simulink model "vehicle_control"  (R2021b)
settings: Solver=ode1  StartTime=0.0  StopTime=Ts  FixedStep=0.01  RelTol=1e-3
values from neighbouring files (symbols this model uses):
  L = 3    [MultiAgent_initiateSAC.m]    (also in control_velocity.m; initiate.m; initiateHybrid.m; initiateSAC.m)
  ld = 5    [MultiAgent_initiateSAC.m]    (also in control_velocity.m; initiate.m = vel/2; initiateHybrid.m; initiateSAC.m)
  psi_o = 0    [MultiAgent_initiateSAC.m]    (also in control_velocity.m; initiate.m; initiateHybrid.m = thetaRefs(1)*(pi/180); initiateSAC.m)
  Ts = 100    [MultiAgent_initiateSAC.m]    (also in control_velocity.m; initiate.m = 30; initiateHybrid.m = 50; initiateSAC.m)
  vel = 5    [MultiAgent_initiateSAC.m]    (also in control_velocity.m = 7; initiate.m = randi([1,10],1,1); initiateHybrid.m; initiateSAC.m)
  X_o = refPose(1,1)+0    [MultiAgent_initiateSAC.m]    (also in control_velocity.m; initiate.m = refPose(1,1)-10; initiateHybrid.m = xRef(1); initiateSAC.m)
  xRef = refPose(:,1)    [MultiAgent_initiateSAC.m]    (also in control_velocity.m; initiate.m; initiateHybrid.m; initiateSAC.m)
  Y_o = -refPose(1,2)+20    [MultiAgent_initiateSAC.m]    (also in control_velocity.m = -refPose(1,2)+0; initiate.m = -refPose(1,2)+10; initiateHybrid.m = yRef(1); initiateSAC.m = -refPose(1,2)+0)
  yRef = -refPose(:,2)    [MultiAgent_initiateSAC.m]    (also in control_velocity.m; initiate.m; initiateHybrid.m; initiateSAC.m)
undefined symbols (not defined in the file or in its folder): DiscIntNeverNeededParam
libraries: vehdynlibviscommon x1, robotalgslib x1, rllib x1, autolibshared x1
settings Model: Creator=berka  LastModifiedBy=berka

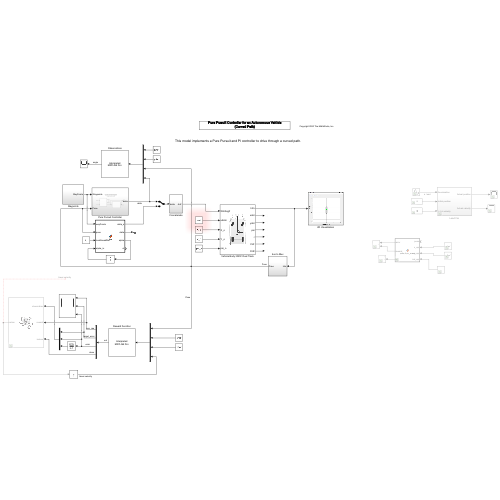
[thumbnail: Simulink's stored preview of the top-level diagram]
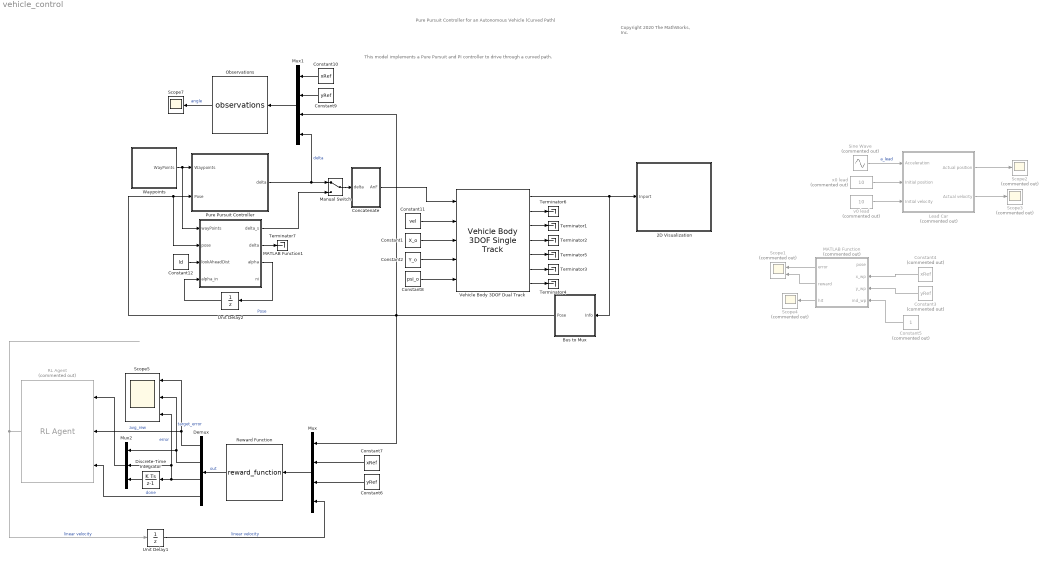
== system vehicle_control ==
  note: Copyright 2020 The MathWorks, Inc.
  note: This model implements a Pure Pursuit and PI controller to drive through a curved path.
  note: Pure Pursuit Controller for an Autonomous Vehicle
      | (Curved Path)
  2D Visualization : Subsystem
      mask Display: image("visualization.JPG");
  Bus to Mux : Subsystem
  Concatenate : Subsystem
  Constant1 : Constant  Value=X_o
  Constant10 : Constant  Value=xRef
  Constant11 : Constant  Value=vel
  Constant12 : Constant  Value=ld
  Constant2 : Constant  Value=Y_o
  Constant3 : Constant  Commented=on  Value=yRef
  Constant4 : Constant  Commented=on  Value=xRef
  Constant5 : Constant  Commented=on
  Constant6 : Constant  Value=yRef
  Constant7 : Constant  Value=xRef
  Constant8 : Constant  Value=psi_o
  Constant9 : Constant  Value=yRef
  Demux : Demux
  Discrete-Time Integrator : DiscreteIntegrator  SampleTime=-1  ICPrevOutput=DiscIntNeverNeededParam  ICPrevScaledInput=DiscIntNeverNeededParam
  Lead Car : Subsystem  Commented=on
  MATLAB Function : MATLAB Function  Commented=on  TreatAsAtomicUnit=on
  MATLAB Function1 : MATLAB Function  TreatAsAtomicUnit=on
  Manual Switch : ManualSwitch
  Mux : Mux
  Mux1 : Mux
  Mux2 : Mux  Inputs=3
  Observations : MATLABFcn  MATLABFcn=observations
  Pure Pursuit Controller : Subsystem
  RL Agent : rllib/RL Agent  Commented=on  Agent=agentObj  ExternalActionAsInput=off  ProvideCumRwd=off  TreatAsDirectFeedthrough=on
  Reward Function : MATLABFcn  MATLABFcn=reward_function
  Scope1 : Scope  Commented=on  NumInputPorts=2
  Scope2 : Scope  Commented=on
  Scope3 : Scope  Commented=on
  Scope4 : Scope  Commented=on
  Scope5 : Scope  NumInputPorts=3
  Scope7 : Scope
  Sine Wave : Sin  Commented=on  Amplitude=0.6  Frequency=0.2  SampleTime=1
  Terminator{1..7} (7 alike) : Terminator
  Unit Delay1 : UnitDelay  SampleTime=-1  HasFrameUpgradeWarning=on
  Unit Delay2 : UnitDelay  SampleTime=-1  HasFrameUpgradeWarning=on
  Vehicle Body 3DOF Dual Track : autolibshared/Vehicle Body 3DOF Single Track  trackMode=Dual  inputMode=External longitudinal velocity  frontSteerMode=on  rearSteerMode=off  windMode=off  muMode=off  extFMode=off  extMMode=off  htchFMode=off  htchMMode=off  extXo=on  extpsio=on  extxdoto=off  extro=off  extYo=on  extTamb=off  extydoto=off  aMode=2  NF=2  NR=2  m=2000  a=1.4  b=1.6  h=0.35  dh=1  hh=0.2  X_o=0  xdot_o=0  CalphaMode=off  sigmaMode=on  d=0  hl=0  w=[1.4,1.4]  Cy_f=12e3  Cy_r=11e3  sigma_f=.1  sigma_r=.1  alpha_f_brk=[-.1 .1]  Cy_f_data=[-9e3 9e3]  alpha_r_brk=[-.1 .1]  Cy_r_data=[-9e3 9e3]  Y_o=0  ydot_o=0  Izz=4000  psi_o=0  r_o=0  Af=2  Cd=.3  Cl=.1  Cpm=.1  beta_w=[0:0.01:0.3]  Cs=[0:0.03:0.9]  Cym=[0:0.01:0.3]  Pabs=101325  Tair=273  g=9.81  mu=1  xdot_tol=.01  Fznom=5000  Fxtire_sat=7e4  Fytire_sat=7e4  longOff=0  latOff=0  vertOff=0  wrapAng=off
      settings: SourceProductBaseCode=PW,DR,MT,UV,VE
  Waypoints : Subsystem
  v0 lead : Constant  Commented=on  Value=10  SampleTime=Ts
  x0 lead : Constant  Commented=on  Value=10  SampleTime=Ts
  wires:
  Vehicle Body 3DOF Dual Track/2 -> Terminator6/1
  Constant1/1 -> Vehicle Body 3DOF Dual Track/3
  Vehicle Body 3DOF Dual Track/3 -> Terminator1/1
  Vehicle Body 3DOF Dual Track/1 -> 2D Visualization/1(Inport), Bus to Mux/1(Info)
  Constant8/1 -> Vehicle Body 3DOF Dual Track/5
  Concatenate/1(AnF) -> Vehicle Body 3DOF Dual Track/1
  Vehicle Body 3DOF Dual Track/6 -> Terminator3/1
  Pure Pursuit Controller/1(delta) -> Manual Switch/1, Mux1/4  "delta"
  Constant2/1 -> Vehicle Body 3DOF Dual Track/4
  Vehicle Body 3DOF Dual Track/7 -> Terminator4/1
  Vehicle Body 3DOF Dual Track/4 -> Terminator2/1
  v0 lead/1 -> Lead Car/3(Initial velocity)
  x0 lead/1 -> Lead Car/2(Initial position)
  Sine Wave/1 -> Lead Car/1(Acceleration)  "a_lead"
  Lead Car/1(Actual position) -> Scope2/1
  Lead Car/2(Actual velocity) -> Scope3/1
  Vehicle Body 3DOF Dual Track/5 -> Terminator5/1
  Waypoints/1(WayPoints) -> MATLAB Function1/1(wayPoints), Pure Pursuit Controller/1(Waypoints)
  Constant4/1 -> MATLAB Function/2(x_wp)
  Constant3/1 -> MATLAB Function/3(y_wp)
  MATLAB Function/1(error) -> Scope1/1
  MATLAB Function/2(reward) -> Scope1/2
  MATLAB Function/3(hit) -> Scope4/1
  Constant5/1 -> MATLAB Function/4(ind_wp)
  Constant6/1 -> Mux/3
  Constant7/1 -> Mux/2
  Mux/1 -> Reward Function/1
  Bus to Mux/1(Pose) -> Mux1/3, MATLAB Function1/2(pose), Pure Pursuit Controller/2(Pose), Mux/1  "Pose"
  Mux1/1 -> Observations/1
  Constant10/1 -> Mux1/1
  Constant9/1 -> Mux1/2
  Observations/1 -> Scope7/1  "angle"
  Reward Function/1 -> Demux/1  "out"
  Demux/1 -> Scope5/1, RL Agent/2  "avg_rew"
  Demux/2 -> Scope5/2, Mux2/1  "target_error"
  Demux/3 -> Scope5/3, Mux2/2, Discrete-Time Integrator/1  "error"
  Discrete-Time Integrator/1 -> Mux2/3
  Mux2/1 -> RL Agent/1
  RL Agent/1 -> Unit Delay1/1  "linear velocity"
  Unit Delay1/1 -> Mux/4  "linear velocity"
  Constant11/1 -> Vehicle Body 3DOF Dual Track/2
  Demux/4 -> RL Agent/3  "done"
  Manual Switch/1 -> Concatenate/1(delta)
  MATLAB Function1/1(delta_s) -> Manual Switch/2
  MATLAB Function1/2(delta) -> Terminator7/1
  Constant12/1 -> MATLAB Function1/3(lookAheadDist)
  MATLAB Function1/3(alpha) -> Unit Delay2/1
  Unit Delay2/1 -> MATLAB Function1/4(alpha_in)

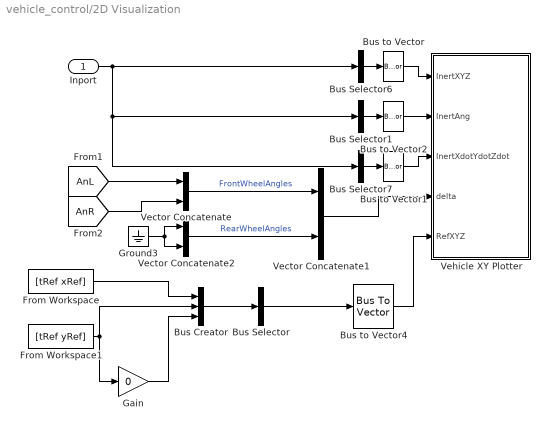
== system vehicle_control/2D Visualization ==
  Inport : Inport
  Bus Creator : BusCreator  Inputs=3
  Bus Selector : BusSelector  OutputSignals=signal1,signal2,signal3  OutputAsBus=on
  Bus Selector1 : BusSelector  OutputSignals=InertFrm.Cg.Ang.phi,InertFrm.Cg.Ang.theta,InertFrm.Cg.Ang.psi  OutputAsBus=on
  Bus Selector6 : BusSelector  OutputSignals=InertFrm.Geom.Disp.X,InertFrm.Geom.Disp.Y,InertFrm.Geom.Disp.Z  OutputAsBus=on
  Bus Selector7 : BusSelector  OutputSignals=InertFrm.Geom.Vel.Xdot,InertFrm.Geom.Vel.Ydot,InertFrm.Geom.Vel.Zdot  OutputAsBus=on
  Bus to Vector{,1..2,4} (4 alike) : BusToVector
  From Workspace : FromWorkspace  VariableName=[tRef xRef]
  From Workspace1 : FromWorkspace  VariableName=[tRef yRef]
  Gain : Gain  Gain=0
  Ground3 : Ground
  Vector Concatenate : Concatenate
  Vector Concatenate1 : Concatenate
  Vector Concatenate2 : Concatenate
  Vehicle XY Plotter : Subsystem  mask(Vehicle XY Plotter){a=2, b=2, w=2, figBorder=10, bufferSize=1024, extRef=on, pltDT=.2}
      mask prompts: a "Distance to front axle from CG, a [m]:"; b "Distance to rear axle from CG, b [m]:"; w "Track width, w [m]:"; figBorder "Distance to figure borders, figBorder [m]:"; bufferSize "Path buffer sampe size, bufferSize []:"; extRef "Plot path reference, extRef"; pltDT "Plot update rate, pltDT [s]:"
      mask help:
      | This block will display a MATLAB figure which indicates the vehicle path, current position and heading velocity.
      | An optional path reference is also provided.
      mask init:
      | if autoblkschecksimstopped(gcb)
      |     PortName = 'RefXYZ';
      |     InportOption  = {'built-in/Ground', [PortName, ' Ground'];...
      |         'built-in/Inport',PortName };
      |     if ~strcmp(get_param(gcb,'extRef'),'on')
      |         NewBlkHdl = autoblksreplaceblock(gcb, InportOption, 1);
      |         set_param(NewBlkHdl, 'ShowName', 'off');
      |     else
      |         autoblksreplaceblock(gcb, InportOption, 2);
      |     end
      | end
      mask TypeOptions a: Vehicle XY Plotter/a
      mask TypeOptions b: Vehicle XY Plotter/b
      mask TypeOptions w: Vehicle XY Plotter/w
      mask TypeOptions figBorder: Vehicle XY Plotter/figBorder
      mask TypeOptions bufferSize: Vehicle XY Plotter/bufferSize
  wires:
  Vector Concatenate1/1 -> Vehicle XY Plotter/4(delta)
  Ground3/1 -> Vector Concatenate2/1, Vector Concatenate2/2
  Bus Selector6/1 -> Bus to Vector/1
  Vector Concatenate/1 -> Vector Concatenate1/1  "FrontWheelAngles"
  [AnL] -> Vector Concatenate/1
  Vector Concatenate2/1 -> Vector Concatenate1/2  "RearWheelAngles"
  Bus Selector7/1 -> Bus to Vector1/1
  Bus to Vector1/1 -> Vehicle XY Plotter/3(InertXdotYdotZdot)
  Bus to Vector/1 -> Vehicle XY Plotter/1(InertXYZ)
  Bus to Vector2/1 -> Vehicle XY Plotter/2(InertAng)
  Bus Selector1/1 -> Bus to Vector2/1
  [AnR] -> Vector Concatenate/2
  Inport/1 -> Bus Selector7/1, Bus Selector1/1, Bus Selector6/1
  Bus to Vector4/1 -> Vehicle XY Plotter/5(RefXYZ)
  Bus Selector/1 -> Bus to Vector4/1
  From Workspace1/1 -> Gain/1, Bus Creator/2
  Gain/1 -> Bus Creator/3
  From Workspace/1 -> Bus Creator/1
  Bus Creator/1 -> Bus Selector/1

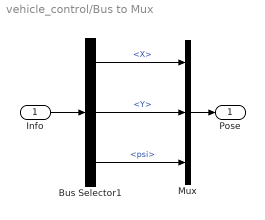
== system vehicle_control/Bus to Mux ==
  Info : Inport
  Bus Selector1 : BusSelector  OutputSignals=InertFrm.Cg.Disp.X,InertFrm.Cg.Disp.Y,InertFrm.Cg.Ang.psi
  Mux : Mux  Inputs=3
  Pose : Outport
  wires:
  Bus Selector1/3 -> Mux/3  "<psi>"
  Bus Selector1/1 -> Mux/1  "<X>"
  Mux/1 -> Pose/1
  Bus Selector1/2 -> Mux/2  "<Y>"
  Info/1 -> Bus Selector1/1

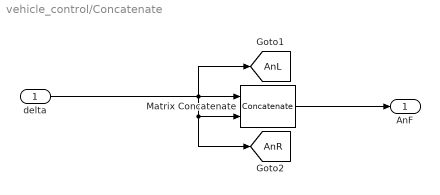
== system vehicle_control/Concatenate ==
  delta : Inport
  Matrix Concatenate : Concatenate
  AnF : Outport  VectorParamsAs1DForOutWhenUnconnected=off
  tag scope: AnL=global, AnR=global
  wires:
  Matrix Concatenate/1 -> AnF/1
  delta/1 -> [AnL], [AnR], Matrix Concatenate/2, Matrix Concatenate/1

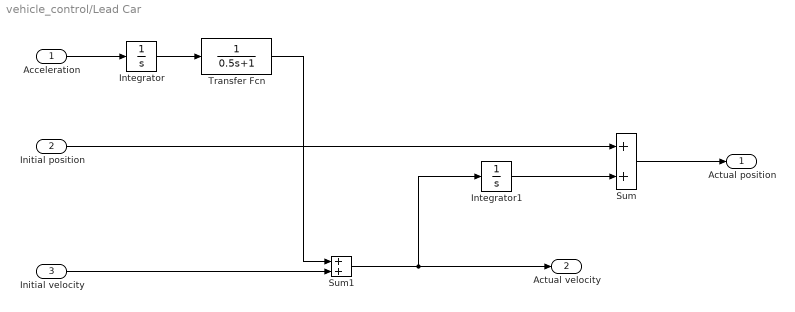
== system vehicle_control/Lead Car ==
  Acceleration : Inport
  Initial position : Inport  Port=2
  Initial velocity : Inport  Port=3
  Integrator : Integrator
  Integrator1 : Integrator
  Sum : Sum
  Sum1 : Sum
  Transfer Fcn : TransferFcn  Denominator=[0.5 1]
  Actual position : Outport  VectorParamsAs1DForOutWhenUnconnected=off
  Actual velocity : Outport  Port=2  VectorParamsAs1DForOutWhenUnconnected=off
  wires:
  Transfer Fcn/1 -> Sum1/1
  Initial velocity/1 -> Sum1/2
  Sum/1 -> Actual position/1
  Integrator/1 -> Transfer Fcn/1
  Sum1/1 -> Integrator1/1, Actual velocity/1
  Acceleration/1 -> Integrator/1
  Initial position/1 -> Sum/1
  Integrator1/1 -> Sum/2

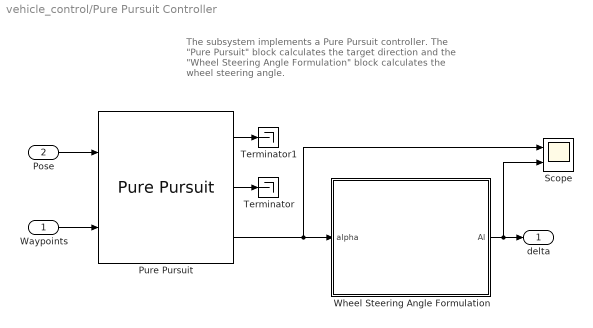
== system vehicle_control/Pure Pursuit Controller ==
  note: The subsystem implements a Pure Pursuit controller. The "Pure Pursuit" block calculates the target direction and the "Wheel Steering Angle Formulation" block calculates the wheel steering angle.
  Waypoints : Inport
  Pose : Inport  Port=2
  Pure Pursuit : robotalgslib/Pure Pursuit  DesiredLinearVelocity=vel  MaxAngularVelocity=1.0  LookaheadDistance=ld  TargetDirPort=on  SimulateUsing=Code generation
  Scope : Scope  NumInputPorts=2
  Terminator : Terminator
  Terminator1 : Terminator
  Wheel Steering Angle Formulation : Subsystem  mask{L=L, ld=ld}
      mask prompts: L "Bicycle length"; ld "Lookahead distance"
      mask TypeOptions L: Bicycle length/Value
      mask TypeOptions ld: Lookahead distance/Value
      mask Display:
      | image("GeometryMask.png")
      | port_label('input', 1, 'alpha')
      | port_label('output', 1, 'delta')
  delta : Outport
  wires:
  Wheel Steering Angle Formulation/1(Al) -> Scope/2, delta/1
  Pure Pursuit/3 -> Scope/1, Wheel Steering Angle Formulation/1(alpha)
  Waypoints/1 -> Pure Pursuit/2
  Pose/1 -> Pure Pursuit/1
  Pure Pursuit/1 -> Terminator1/1
  Pure Pursuit/2 -> Terminator/1

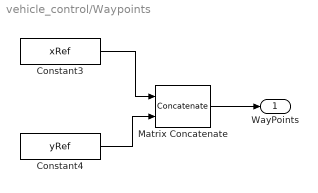
== system vehicle_control/Waypoints ==
  Constant3 : Constant  Value=xRef  SampleTime=0.1
  Constant4 : Constant  Value=yRef  SampleTime=0.1
  Matrix Concatenate : Concatenate  Mode=Multidimensional array  ConcatenateDimension=2
  WayPoints : Outport
  wires:
  Constant4/1 -> Matrix Concatenate/2
  Matrix Concatenate/1 -> WayPoints/1
  Constant3/1 -> Matrix Concatenate/1

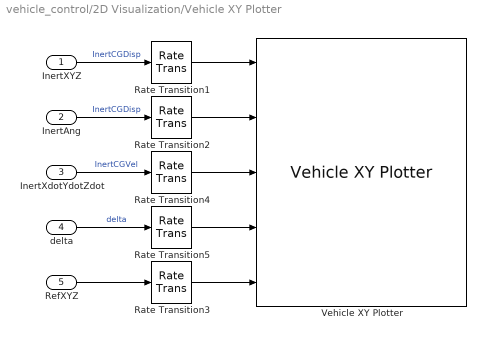
== system vehicle_control/2D Visualization/Vehicle XY Plotter ==
  InertXYZ : Inport
  InertAng : Inport  Port=2
  InertXdotYdotZdot : Inport  Port=3
  delta : Inport  Port=4
  RefXYZ : Inport  Port=5
  Rate Transition{1..5} (5 alike) : RateTransition  Deterministic=off  OutPortSampleTime=pltDT
  Vehicle XY Plotter : vehdynlibviscommon/Vehicle XY Plotter  w=w  a=a  b=b  figBorder=figBorder  bufferSize=bufferSize  extStats=off  extTireF=off
      settings: SourceProductBaseCode=VE
  wires:
  Rate Transition5/1 -> Vehicle XY Plotter/4
  Rate Transition4/1 -> Vehicle XY Plotter/3
  Rate Transition2/1 -> Vehicle XY Plotter/2
  Rate Transition1/1 -> Vehicle XY Plotter/1
  Rate Transition3/1 -> Vehicle XY Plotter/5
  delta/1 -> Rate Transition5/1  "delta"
  InertXYZ/1 -> Rate Transition1/1  "InertCGDisp"
  InertXdotYdotZdot/1 -> Rate Transition4/1  "InertCGVel"
  InertAng/1 -> Rate Transition2/1  "InertCGDisp"
  RefXYZ/1 -> Rate Transition3/1

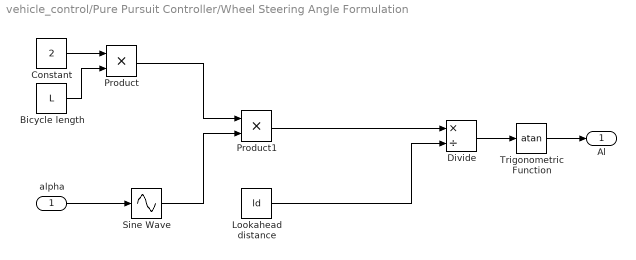
== system vehicle_control/Pure Pursuit Controller/Wheel Steering Angle Formulation ==
  alpha : Inport
  Bicycle length : Constant  Value=L
  Constant : Constant  Value=2
  Divide : Product  Inputs=*/
  Lookahead distance : Constant  Value=ld
  Product : Product
  Product1 : Product
  Sine Wave : Sin  TimeSource=Use external signal  SampleTime=0
  Trigonometric Function : Trigonometry  Operator=atan
  Al : Outport
  wires:
  Sine Wave/1 -> Product1/2
  Bicycle length/1 -> Product/2
  Constant/1 -> Product/1
  Product1/1 -> Divide/1
  Product/1 -> Product1/1
  Divide/1 -> Trigonometric Function/1
  Trigonometric Function/1 -> Al/1
  alpha/1 -> Sine Wave/1
  Lookahead distance/1 -> Divide/2

== matlab function vehicle_control/MATLAB Function1 ==
  data: delta_s output; wayPoints input; delta output; pose input; lookAheadDist input; alpha_in input; alpha output; ni output
function [delta_s, delta, alpha, ni] = fcn(wayPoints, pose, lookAheadDist,alpha_in)

% Pure Pursuit Configuration Parameters

L = 3; % Vehicle length
max_angVel = 1;
smp = 0.01; % sampling time


% Vehicle Pose
x = pose(1);
y = pose(2);
psi = pose(3);

dx = abs(x - wayPoints(:,1));  % distance to all waypoints at the current time
dy = abs(y - wayPoints(:,2));

lp = hypot(dx, dy); %Find hypotenuse 

[sWayPoints, idx] = sort(lp); % sort the way points according to distance



ni = idx(1); % nearest point candidate

for i=1:1:length(idx)-1

    % check for forward direction
    tx = wayPoints(idx(i),1); 
    ty = wayPoints(idx(i),2);
    
    d_angle = atan2((ty-y),(tx-x)); % direction angle

    if (d_angle>deg2rad(-90) && d_angle<deg2rad(90))
        ni = idx(i); % nearest next waypoint index
        break;
    end

end
while lookAheadDist >= lp(ni)

    ni = ni + 1;

    if (ni >= length(wayPoints(:,1)))
        break;
    end

end

if ni==16
    ni = 15;
end
tx = wayPoints(ni,1); 
ty = wayPoints(ni,2);

d_angle = atan2((ty-y),(tx-x)); % direction angle

alpha = (d_angle - psi);

% if (alpha - alpha_in)/smp > max_angVel
%     alpha = alpha_in + smp*max_angVel;
% end

delta = 2*sin(alpha)/lookAheadDist; % for non-steering vehicles ex: drones

delta_s = 0.5*atan(2*L*sin(alpha)/lookAheadDist);

end

== matlab function vehicle_control/MATLAB Function ==
  data: pose input; error output; x_wp input; y_wp input; reward output; ind_wp input; hit output
function [error, reward, hit]  = calculate_error(pose,x_wp,y_wp,ind_wp)
    threshold = 0.5;
    reward = 0;
    hit = 0;

    x_pos = pose(1);
    y_pos = pose(2);
    theta = pose(3);
    
    error = sqrt((x_wp(ind_wp)-x_pos)^2 + (y_wp(ind_wp)-y_pos)^2);
    if error<threshold
        reward = reward + 10;
        hit =1;
    end

end
